simulink model "Modelesimulink_l2p2"  (Simulink 8.7)
settings: Solver=ode3  StartTime=0.0  StopTime=0.001  FixedStep=0.0001  RelTol=1e-3
values from neighbouring files (symbols this model uses):
  Ctilde = diag(diag(Neolambda'.*C.*Neolambda))    [labo2p1.m]
  Imod = diag(diag(Neolambda'*M*Neolambda))    [labo2p1.m]
  phi = [0;0;-2.77;0]    [labo2p1.m]
  R = Neolambda'*F    [labo2p1.m]
  V = NeoPhi    [labo2p1.m]
  wombo = 48.48    [labo2p1.m]
settings Model: Creator=p202400  LastModifiedBy=sitanb
settings DataIOCC: SignalLoggingSaveFormat=ModelDataLogs
settings OptimizationCC: ExpressionDepthLimit=2147483647
settings DebuggingCC: SolverPrmCheckMsg=warning  FcnCallInpInsideContextMsg=UseLocalSettings  StateNameClashWarn=warning
settings GRTTargetCC: CombineOutputUpdateFcns=off  GRTInterface=on

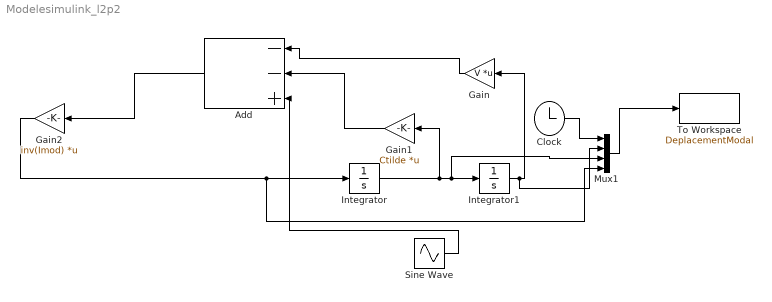
== system Modelesimulink_l2p2 ==
  Add : Sum  Inputs=--+
  Clock : Clock
  Gain : Gain  Gain=V  Multiplication=Matrix(K*u) (u vector)
  Gain1 : Gain  Gain=Ctilde  Multiplication=Matrix(K*u) (u vector)
  Gain2 : Gain  Gain=inv(Imod)  Multiplication=Matrix(K*u) (u vector)
  Integrator : Integrator
  Integrator1 : Integrator
  Mux1 : Mux
  Sine Wave : Sin  Amplitude=R  Frequency=wombo  Phase=phi  SampleTime=0
  To Workspace : ToWorkspace  VariableName=DeplacementModal  SampleTime=-1
  wires:
  Integrator/1 -> Mux1/3, Integrator1/1, Gain1/1
  Integrator1/1 -> Gain/1, Mux1/2
  Gain1/1 -> Add/2
  Gain/1 -> Add/1
  Clock/1 -> Mux1/1
  Mux1/1 -> To Workspace/1
  Sine Wave/1 -> Add/3
  Gain2/1 -> Mux1/4, Integrator/1
  Add/1 -> Gain2/1
